simulink model "FSMC_sim"  (R2020a)
settings: Solver=VariableStepAuto  StartTime=0.0  StopTime=10.0  RelTol=1e-3
settings Model: Creator=Tomy  LastModifiedBy=Tomy

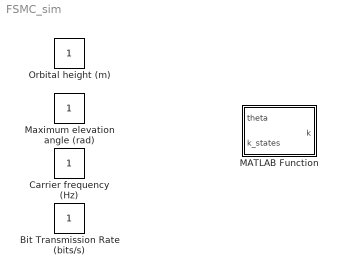
== system FSMC_sim ==
  Bit Transmission Rate (bits/s) : Constant
  Carrier frequency (Hz) : Constant
  MATLAB Function : MATLAB Function  TreatAsAtomicUnit=on
  Maximum elevation angle (rad) : Constant
  Orbital height (m) : Constant

== matlab function FSMC_sim/MATLAB Function ==
  data: theta input; k output; k_states input
function k = FSMC_parameters(theta, k_states)

k = theta;
